simulink model "buttonblink_task"  (Simulink 3.00)
libraries: genlib x2, mathlib x2, logiclib x1

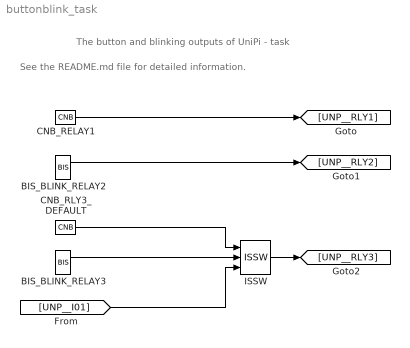
== system buttonblink_task ==
  note: See the README.md file for detailed information.
  note: The button and blinking outputs of UniPi - task
  BIS_BLINK_RELAY2 : genlib/BIS  Y0=off  t1=1  t2=2  t3=0  t4=4  t5=5  t6=6  t7=7  t8=8  RPT=on  bEdit=off
  BIS_BLINK_RELAY3 : genlib/BIS  Y0=off  t1=0.2  t2=0.4  t3=0  t4=0  t5=0  t6=0  t7=2.0  t8=0  RPT=on  bEdit=off
  CNB_RELAY1 : mathlib/CNB  YCN=on
  CNB_RLY3_DEFAULT : mathlib/CNB  YCN=off
  ISSW : logiclib/ISSW
  wires:
  BIS_BLINK_RELAY2/1 -> [UNP__RLY2]
  BIS_BLINK_RELAY3/1 -> ISSW/2
  CNB_RELAY1/1 -> [UNP__RLY1]
  CNB_RLY3_DEFAULT/1 -> ISSW/1
  [UNP__I01] -> ISSW/3
  ISSW/1 -> [UNP__RLY3]
